simulink model "LCK"  (R2018b)
settings: Solver=FixedStepDiscrete  StartTime=0.0  StopTime=inf  FixedStep=0.01  RelTol=1e-3
PostLoadFcn:
  | if any(exist('dsrtsu_mdlpostloadfcn', 'file') ~= 0), dsrtsu_mdlpostloadfcn('Execute', bdroot); end
values from neighbouring files (symbols this model uses):
  C_DEG2RAD = 0.0175    [LCK_Macro.sldd]
  C_KPH2MPS = 0.2778    [LCK_Macro.sldd]
  C_NEARZERO = 0.0001    [LCK_Macro.sldd]
  C_ONE = 1.0    [LCK_Macro.sldd]
  C_RAD2DEG = 57.2958    [LCK_Macro.sldd]
  C_ZERO = 0.0    [LCK_Macro.sldd]
  k_accel_pedal_pos_per_speed_x : value not decoded    [LCK_LogicPara.sldd]
  k_accel_pedal_pos_per_speed_z : value not decoded    [LCK_LogicPara.sldd]
  k_brake_suprress_hold = 1000.0    [LCK_LogicPara.sldd]
  k_driver_appl_torque_filt = 50.0    [LCK_LogicPara.sldd]
  k_driver_suppression_hold_time = 3000.0    [LCK_LogicPara.sldd]
  k_hands_on_wheel_hold_msec = 500.0    [LCK_LogicPara.sldd]
  k_hands_on_wheel_torque_hi = 0.2    [LCK_LogicPara.sldd]
  k_hands_on_wheel_torque_lo = 0.15    [LCK_LogicPara.sldd]
  k_handsoff_delay_cycles = 50.0    [LCK_LogicPara.sldd]
  k_handsoff_torq_Lo_CR = 0.3    [LCK_LogicPara.sldd]
  k_handson_delay_cycles = 5.0    [LCK_LogicPara.sldd]
  k_HighAccel_suppress_hold = 3000.0    [LCK_LogicPara.sldd]
  k_HLR_suprress_hold = 3000.0    [LCK_LogicPara.sldd]
  k_hs_StrAng_CR_threshold_z : value not decoded    [LCK_LogicPara.sldd]
  k_LC_Exit_Switch = 0.0    [LCK_LogicPara.sldd]
  k_LCG_Configured = 1.0    [LCK_LogicPara.sldd]
  k_LCK_A0_Rdy2Act_UseConst = 0.0    [LCK_LogicPara.sldd]
  k_LCK_A0Fac_ActSta : value not decoded    [LCK_CtrlPara.sldd]
  k_LCK_A0Fac_DrvStm : value not decoded    [LCK_CtrlPara.sldd]
  k_LCK_A0Shift_LftCurv : value not decoded    [LCK_CtrlPara.sldd]
  k_LCK_A0Shift_RgtCurv : value not decoded    [LCK_CtrlPara.sldd]
  k_LCK_A0Shift_StraLan = 0.0    [LCK_CtrlPara.sldd]
  k_LCK_A0ShiftFac_Dy_LftCurv : value not decoded    [LCK_CtrlPara.sldd]
  k_LCK_A0ShiftFac_Dy_RgtCurv : value not decoded    [LCK_CtrlPara.sldd]
  k_LCK_A0ShiftFac_Vspd : value not decoded    [LCK_CtrlPara.sldd]
  k_LCK_accel_inhibit_thold = 35.0    [LCK_LogicPara.sldd]
  k_LCK_Active2Ready_Mask = 255.0    [LCK_LogicPara.sldd]
  k_LCK_CvatRateBks : value not decoded    [LCK_CtrlPara.sldd]
  k_LCK_CvatrBks : value not decoded    [LCK_CtrlPara.sldd]
  k_LCK_DFac_Dy : value not decoded    [LCK_CtrlPara.sldd]
  k_LCK_DFac_Dy_Curv : value not decoded    [LCK_CtrlPara.sldd]
  k_LCK_DFac_HaCurCen : value not decoded    [LCK_CtrlPara.sldd]
  k_LCK_DFac_HaCurSid : value not decoded    [LCK_CtrlPara.sldd]
  k_LCK_DFac_HadCurCen : value not decoded    [LCK_CtrlPara.sldd]
  k_LCK_DFac_HadCurSid : value not decoded    [LCK_CtrlPara.sldd]
  k_LCK_DFac_HadStrCen : value not decoded    [LCK_CtrlPara.sldd]
  k_LCK_DFac_HadStrSid : value not decoded    [LCK_CtrlPara.sldd]
  k_LCK_DFac_HaStrCen : value not decoded    [LCK_CtrlPara.sldd]
  k_LCK_DFac_HaStrSid : value not decoded    [LCK_CtrlPara.sldd]
  k_LCK_DFac_Rad : value not decoded    [LCK_CtrlPara.sldd]
  k_LCK_DFac_SA_CurCen : value not decoded    [LCK_CtrlPara.sldd]
  k_LCK_DFac_SA_CurSid : value not decoded    [LCK_CtrlPara.sldd]
  k_LCK_DFac_SA_StrCen : value not decoded    [LCK_CtrlPara.sldd]
  k_LCK_DFac_SA_StrSid : value not decoded    [LCK_CtrlPara.sldd]
  k_LCK_DFac_SS_CurCen : value not decoded    [LCK_CtrlPara.sldd]
  k_LCK_DFac_SS_CurSid : value not decoded    [LCK_CtrlPara.sldd]
  k_LCK_DFac_SS_StrCen : value not decoded    [LCK_CtrlPara.sldd]
  k_LCK_DFac_SS_StrSid : value not decoded    [LCK_CtrlPara.sldd]
  k_LCK_DFac_Vspd : value not decoded    [LCK_CtrlPara.sldd]
  k_LCK_DlyTm_DrvStim = 0.2    [LCK_CtrlPara.sldd]
  k_LCK_DTermMax = 2.0    [LCK_CtrlPara.sldd]
  k_LCK_DyBks_Curv : value not decoded    [LCK_CtrlPara.sldd]
  k_LCK_Enable_POOnly = 1.0    [LCK_LogicPara.sldd]
  k_LCK_Entry_DistBuffer = 0.1    [LCK_LogicPara.sldd]
  k_LCK_Fac_Vspd2RngThr_FalRec = 0.23    [LCK_CtrlPara.sldd]
  k_LCK_Ffw_CvatSwh = 0.0    [LCK_CtrlPara.sldd]
  k_LCK_Ffw_DyBks : value not decoded    [LCK_CtrlPara.sldd]
  k_LCK_Ffw_TimCon_CmdFlt = 0.0    [LCK_CtrlPara.sldd]
  k_LCK_FfwDeltaFac_Rad_Lft : value not decoded    [LCK_CtrlPara.sldd]
  k_LCK_FfwDeltaFac_Rad_Rgt : value not decoded    [LCK_CtrlPara.sldd]
  k_LCK_FfwDeltaFac_Vspd : value not decoded    [LCK_CtrlPara.sldd]
  k_LCK_FfwFac_CvatRate_Lft : value not decoded    [LCK_CtrlPara.sldd]
  k_LCK_FfwFac_CvatRate_Rgt : value not decoded    [LCK_CtrlPara.sldd]
  k_LCK_FfwFac_Dy : value not decoded    [LCK_CtrlPara.sldd]
  k_LCK_FfwFac_Rad_Lft : value not decoded    [LCK_CtrlPara.sldd]
  k_LCK_FfwFac_Rad_Rgt : value not decoded    [LCK_CtrlPara.sldd]
  k_LCK_FfwFac_Vspd : value not decoded    [LCK_CtrlPara.sldd]
  k_LCK_FfwTorq_Cvat : value not decoded    [LCK_CtrlPara.sldd]
  k_LCK_HAFac_ActSta : value not decoded    [LCK_CtrlPara.sldd]
  k_LCK_HAFac_DrvStm : value not decoded    [LCK_CtrlPara.sldd]
  k_LCK_HaloTime = 2000.0    [LCK_LogicPara.sldd]
  k_LCK_HaloTime_Switch = 0.0    [LCK_LogicPara.sldd]
  k_LCK_HARFac_ActSta : value not decoded    [LCK_CtrlPara.sldd]
  k_LCK_HARFac_DrvStm : value not decoded    [LCK_CtrlPara.sldd]
  k_LCK_Hed_DyBks : value not decoded    [LCK_CtrlPara.sldd]
  k_LCK_HedAngDiffX : value not decoded    [LCK_CtrlPara.sldd]
  k_LCK_HedAngRateDiffX : value not decoded    [LCK_CtrlPara.sldd]
  k_LCK_HndsOnWhel_DlyTm_Idl2Rdy = 0.0    [LCK_LogicPara.sldd]
  k_LCK_host_veh_width = 1.86    [LCK_LogicPara.sldd]
  k_LCK_Idle2Ready_Mask = 239.0    [LCK_LogicPara.sldd]
  k_LCK_Junc_SusTime = 1.0    [LCK_LogicPara.sldd]
  k_LCK_KpKdDecSlopeLmt = 10.0    [LCK_CtrlPara.sldd]
  k_LCK_KpKdIncSlopeLmt = 5.0    [LCK_CtrlPara.sldd]
  k_LCK_Lat_Ctrl_DFac_Lft = 1.0    [LCK_CtrlPara.sldd]
  k_LCK_Lat_Ctrl_DFac_Rgt = 1.05    [LCK_CtrlPara.sldd]
  k_LCK_Lat_Ctrl_Kd = 0.8    [LCK_CtrlPara.sldd]
  k_LCK_Lat_Ctrl_Ki = 0.5    [LCK_CtrlPara.sldd]
  k_LCK_Lat_Ctrl_Kp = 0.7    [LCK_CtrlPara.sldd]
  k_LCK_Lat_Ctrl_Kp_NearGain = 0.7    [LCK_CtrlPara.sldd]
  k_LCK_Lat_Ctrl_PFac_Lft = 1.0    [LCK_CtrlPara.sldd]
  k_LCK_Lat_Ctrl_PFac_Rgt = 1.05    [LCK_CtrlPara.sldd]
  k_LCK_Lat_Ctrl_TimCon_CmdFlt = 5.0    [LCK_CtrlPara.sldd]
  k_LCK_Lat_DFac_Rad : value not decoded    [LCK_CtrlPara.sldd]
  k_LCK_Lat_DFac_SS_Cur : value not decoded    [LCK_CtrlPara.sldd]
  k_LCK_Lat_DFac_SS_Str : value not decoded    [LCK_CtrlPara.sldd]
  k_LCK_Lat_DFac_Vspd : value not decoded    [LCK_CtrlPara.sldd]
  k_LCK_Lat_DyBks : value not decoded    [LCK_CtrlPara.sldd]
  k_LCK_Lat_IFac_Rad : value not decoded    [LCK_CtrlPara.sldd]
  k_LCK_Lat_IFac_Vspd : value not decoded    [LCK_CtrlPara.sldd]
  k_LCK_Lat_ILmtFac_Dy_CurvLan : value not decoded    [LCK_CtrlPara.sldd]
  k_LCK_Lat_ILmtFac_Dy_StraLan : value not decoded    [LCK_CtrlPara.sldd]
  k_LCK_Lat_ILmtFac_Rad : value not decoded    [LCK_CtrlPara.sldd]
  k_LCK_Lat_ILmtFac_Rad_NearGain = 1.0    [LCK_CtrlPara.sldd]
  k_LCK_Lat_ILmtFac_Vspd_CurvLan : value not decoded    [LCK_CtrlPara.sldd]
  k_LCK_Lat_ILmtFac_Vspd_StraLan : value not decoded    [LCK_CtrlPara.sldd]
  k_LCK_Lat_ITermLmt_Dy = 1.0    [LCK_CtrlPara.sldd]
  k_LCK_Lat_KpKdDecSlopeLmt = 10.0    [LCK_CtrlPara.sldd]
  k_LCK_Lat_KpKdIncSlopeLmt = 10.0    [LCK_CtrlPara.sldd]
  k_LCK_Lat_PFac_Dy_InnLftCur : value not decoded    [LCK_CtrlPara.sldd]
  k_LCK_Lat_PFac_Dy_InnRgtCur : value not decoded    [LCK_CtrlPara.sldd]
  k_LCK_Lat_PFac_Dy_OutLftCur : value not decoded    [LCK_CtrlPara.sldd]
  k_LCK_Lat_PFac_Dy_OutRgtCur : value not decoded    [LCK_CtrlPara.sldd]
  k_LCK_Lat_PFac_Dy_Str : value not decoded    [LCK_CtrlPara.sldd]
  k_LCK_Lat_PFac_Rad : value not decoded    [LCK_CtrlPara.sldd]
  ... (+153 more)
undefined symbols (not defined in the file or in its folder): k_LCK_CurvBks, K_LCK_SPA0A1A2_LMRngCmp_y
libraries: LateralControl_fcns_lib x59, simulink x24
(part 25 of 47)

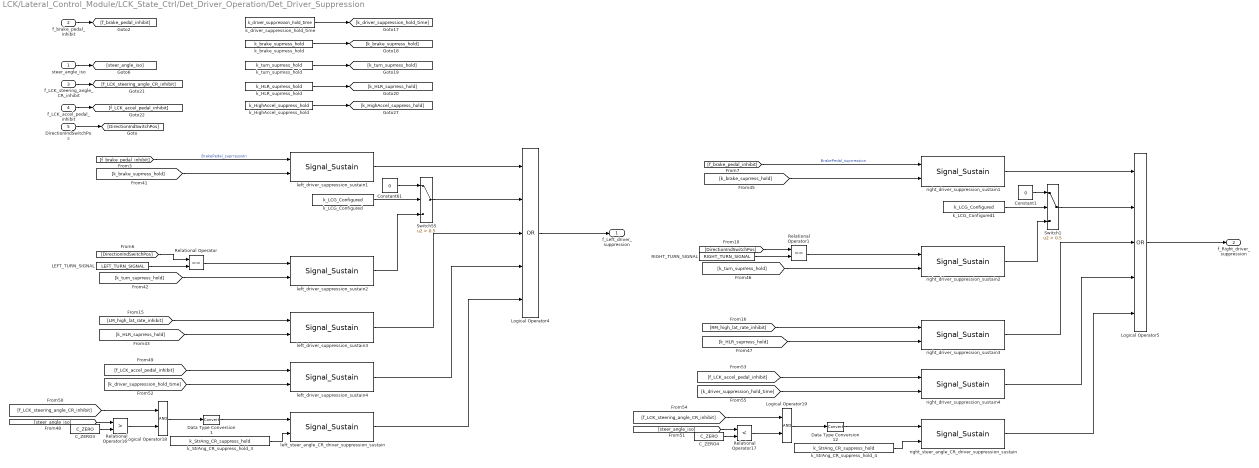
== system LCK/Lateral_Control_Module/LCK_State_Ctrl/Det_Driver_Operation/Det_Driver_Suppression ==
  steer_angle_iso : Inport  Description=_GWMAB30P4.Latctrl.000_62_
  f_brake_pedal_inhibit : Inport  Description=_GWMAB30P4.Latctrl.000_59_  Port=2
  f_LCK_steering_angle_CR_inhibit : Inport  Description=_GACA26P3.Latctrl.000_19_  Port=3
  f_LCK_accel_pedal_inhibit : Inport  Description=_GACA26P3.Latctrl.000_20_  Port=4
  DirectionIndSwitchPos : Inport  Description=_GACA26P3.Latctrl.000_20_  Port=5
  C_ZERO3 : Constant  Description=_GACA26P3.Latctrl.000_21_  Value=C_ZERO
  C_ZERO4 : Constant  Description=_GACA26P3.Latctrl.000_22_  Value=C_ZERO
  Constant1 : Constant  Tag={'output',{'type','Int32'},'date',737462.50906574074}  Description=_GWMH9P4.LCK.000_53_  Value=0
  Constant61 : Constant  Tag={'output',{'type','Int32'},'date',737462.50906574074}  Description=_GWMH9P4.LCK.000_53_  Value=0
  Data Type Conversion1 : DataTypeConversion  Description=_GWMAB30P4.Latctrl.000_70_
  Data Type Conversion12 : DataTypeConversion  Description=_GACA26P3.Latctrl.000_23_
  LEFT_TURN_SIGNAL : Constant  Description=_GWMAB30P3.Latctrl.000_57_  Value=LEFT_TURN_SIGNAL
  Logical Operator18 : Logic  Description=_GACA26P3.Latctrl.000_24_  AllPortsSameDT=off  OutDataTypeStr=boolean
  Logical Operator19 : Logic  Description=_GACA26P3.Latctrl.000_25_  AllPortsSameDT=off  OutDataTypeStr=boolean
  Logical Operator4 : Logic  Description=_GWMAB30P3.Latctrl.000_71_  Operator=OR  Inputs=5  AllPortsSameDT=off  OutDataTypeStr=boolean
  Logical Operator5 : Logic  Description=_GWMAB30P3.Latctrl.000_72_  Operator=OR  Inputs=5  AllPortsSameDT=off  OutDataTypeStr=boolean
  RIGHT_TURN_SIGNAL : Constant  Description=_GWMAB30P3.Latctrl.000_77_  Value=RIGHT_TURN_SIGNAL
  Relational Operator : RelationalOperator  Description=_GWMAB30P3.Latctrl.000_79_  Operator===  OutDataTypeStr=boolean  RndMeth=Nearest
  Relational Operator1 : RelationalOperator  Description=_GWMAB30P3.Latctrl.000_80_  Operator===  OutDataTypeStr=boolean  RndMeth=Nearest
  Relational Operator16 : RelationalOperator  Description=_GACA26P3.Latctrl.000_26_  Operator=>  OutDataTypeStr=boolean  RndMeth=Nearest
  Relational Operator17 : RelationalOperator  Description=_GACA26P3.Latctrl.000_27_  Operator=<  OutDataTypeStr=boolean  RndMeth=Nearest
  Switch1 : Switch  Tag={'output',{'type','Bool'},'threshold',{'type','Int32'},'date',737463.78898939816}  Description=_GWMH9P4.LCK.000_143_  Criteria=u2 > Threshold  Threshold=0.5
  Switch55 : Switch  Tag={'output',{'type','Bool'},'threshold',{'type','Int32'},'date',737463.78898939816}  Description=_GWMH9P4.LCK.000_143_  Criteria=u2 > Threshold  Threshold=0.5
  k_HLR_suprress_hold : Constant  Description=_GACA26P3.Latctrl.000_28_  Value=k_HLR_suprress_hold
  k_HighAccel_suppress_hold : Constant  Description=_GACA26P3.Latctrl.000_28_  Value=k_HighAccel_suppress_hold
  k_LCG_Configured : Constant  Tag={'output',{'name','$P','class','EXTERN_CAL','type','Bool'},'date',737462.72265947913}  Description=_GWMH9P4.LCK.000_170_  Value=k_LCG_Configured
  k_LCG_Configured1 : Constant  Tag={'output',{'name','$P','class','EXTERN_CAL','type','Bool'},'date',737462.72265947913}  Description=_GWMH9P4.LCK.000_170_  Value=k_LCG_Configured
  k_StrAng_CR_suppress_hold_3 : Constant  Description=_GACA26P3.Latctrl.000_29_  Value=k_StrAng_CR_suppress_hold
  k_StrAng_CR_suppress_hold_4 : Constant  Description=_GACA26P3.Latctrl.000_30_  Value=k_StrAng_CR_suppress_hold
  k_brake_suprress_hold : Constant  Description=_GACA26P3.Latctrl.000_31_  Value=k_brake_suprress_hold
  k_driver_suppression_hold_time : Constant  Description=_GWMAB30P3.Latctrl.000_97_  Value=k_driver_suppression_hold_time
  k_turn_suprress_hold : Constant  Description=_GACA26P3.Latctrl.000_32_  Value=k_turn_suprress_hold
  left_driver_suppression_sustain{1..4} (4 alike) : LateralControl_fcns_lib/Signal_Sustain  Description=_GWMAB30P4.LKAFN.000_315_  SystemSampleTime=-1
  left_steer_angle_CR_driver_suppression_sustain : LateralControl_fcns_lib/Signal_Sustain  Description=_GWMAB30P4.LKAFN.000_315_  SystemSampleTime=-1
  right_driver_suppression_sustain{1..4} (4 alike) : LateralControl_fcns_lib/Signal_Sustain  Description=_GWMAB30P4.LKAFN.000_315_  SystemSampleTime=-1
  right_steer_angle_CR_driver_suppression_sustain : LateralControl_fcns_lib/Signal_Sustain  Description=_GWMAB30P4.LKAFN.000_315_  SystemSampleTime=-1
  f_Left_driver_suppression : Outport  Description=_GWMAB30P4.Latctrl.000_95_
  f_Right_driver_suppression : Outport  Description=_GWMAB30P4.Latctrl.000_96_  Port=2
  wires:
  [k_HLR_suprress_hold] -> right_driver_suppression_sustain3/2
  [steer_angle_iso] -> Relational Operator17/1
  [RM_high_lat_rate_inhibit] -> right_driver_suppression_sustain3/1
  right_driver_suppression_sustain1/1 -> Logical Operator5/1
  RIGHT_TURN_SIGNAL/1 -> Relational Operator1/2
  C_ZERO4/1 -> Relational Operator17/2
  Logical Operator5/1 -> f_Right_driver_suppression/1
  [f_LCK_accel_pedal_inhibit] -> right_driver_suppression_sustain4/1
  [DirectionIndSwitchPos] -> Relational Operator1/1
  [k_turn_suprress_hold] -> right_driver_suppression_sustain2/2
  [f_brake_pedal_inhibit] -> right_driver_suppression_sustain1/1  "BrakePedal_suprression"
  [k_driver_suppression_hold_time] -> right_driver_suppression_sustain4/2
  [k_brake_suprress_hold] -> right_driver_suppression_sustain1/2
  Logical Operator19/1 -> Data Type Conversion12/1
  right_driver_suppression_sustain3/1 -> Logical Operator5/3
  Relational Operator1/1 -> right_driver_suppression_sustain2/1
  right_steer_angle_CR_driver_suppression_sustain/1 -> Logical Operator5/5
  [f_LCK_steering_angle_CR_inhibit] -> Logical Operator19/1
  k_StrAng_CR_suppress_hold_4/1 -> right_steer_angle_CR_driver_suppression_sustain/2
  right_driver_suppression_sustain4/1 -> Logical Operator5/4
  Relational Operator17/1 -> Logical Operator19/2
  [k_HLR_suprress_hold] -> left_driver_suppression_sustain3/2
  left_steer_angle_CR_driver_suppression_sustain/1 -> Logical Operator4/5
  C_ZERO3/1 -> Relational Operator16/2
  [f_LCK_steering_angle_CR_inhibit] -> Logical Operator18/1
  LEFT_TURN_SIGNAL/1 -> Relational Operator/2
  Logical Operator18/1 -> Data Type Conversion1/1
  Logical Operator4/1 -> f_Left_driver_suppression/1
  left_driver_suppression_sustain1/1 -> Logical Operator4/1
  [steer_angle_iso] -> Relational Operator16/1
  [f_brake_pedal_inhibit] -> left_driver_suppression_sustain1/1  "BrakePedal_suprression"
  [LM_high_lat_rate_inhibit] -> left_driver_suppression_sustain3/1
  [k_turn_suprress_hold] -> left_driver_suppression_sustain2/2
  [k_brake_suprress_hold] -> left_driver_suppression_sustain1/2
  k_StrAng_CR_suppress_hold_3/1 -> left_steer_angle_CR_driver_suppression_sustain/2
  Relational Operator/1 -> left_driver_suppression_sustain2/1
  left_driver_suppression_sustain4/1 -> Logical Operator4/4
  left_driver_suppression_sustain3/1 -> Logical Operator4/3
  [k_driver_suppression_hold_time] -> left_driver_suppression_sustain4/2
  Data Type Conversion1/1 -> left_steer_angle_CR_driver_suppression_sustain/1
  Relational Operator16/1 -> Logical Operator18/2
  [f_LCK_accel_pedal_inhibit] -> left_driver_suppression_sustain4/1
  [DirectionIndSwitchPos] -> Relational Operator/1
  steer_angle_iso/1 -> [steer_angle_iso]
  f_brake_pedal_inhibit/1 -> [f_brake_pedal_inhibit]
  f_LCK_accel_pedal_inhibit/1 -> [f_LCK_accel_pedal_inhibit]
  f_LCK_steering_angle_CR_inhibit/1 -> [f_LCK_steering_angle_CR_inhibit]
  k_HLR_suprress_hold/1 -> [k_HLR_suprress_hold]
  k_brake_suprress_hold/1 -> [k_brake_suprress_hold]
  k_driver_suppression_hold_time/1 -> [k_driver_suppression_hold_time]
  k_HighAccel_suppress_hold/1 -> [k_HighAccel_suppress_hold]
  k_turn_suprress_hold/1 -> [k_turn_suprress_hold]
  Data Type Conversion12/1 -> right_steer_angle_CR_driver_suppression_sustain/1
  DirectionIndSwitchPos/1 -> [DirectionIndSwitchPos]
  k_LCG_Configured/1 -> Switch55/2
  Switch55/1 -> Logical Operator4/2
  left_driver_suppression_sustain2/1 -> Switch55/3
  Constant61/1 -> Switch55/1
  k_LCG_Configured1/1 -> Switch1/2
  Switch1/1 -> Logical Operator5/2
  right_driver_suppression_sustain2/1 -> Switch1/3
  Constant1/1 -> Switch1/1
